simulink model "MPCsimulation_tuning_2016B"  (R2016b)
settings: Solver=VariableStepAuto  StartTime=0.0  StopTime=30.0  RelTol=1e-3
InitFcn:
  | dynrotpend
undefined symbols (not defined in the file or in its folder): matrcomp, par
libraries: dspinverses x2, mpclib x1, simulink x1
settings Model: Creator=janneke  LastModifiedBy=janneke
settings SFSimCC: SimUseLocalCustomCode=on
settings RTWCC: RTWUseLocalCustomCode=on

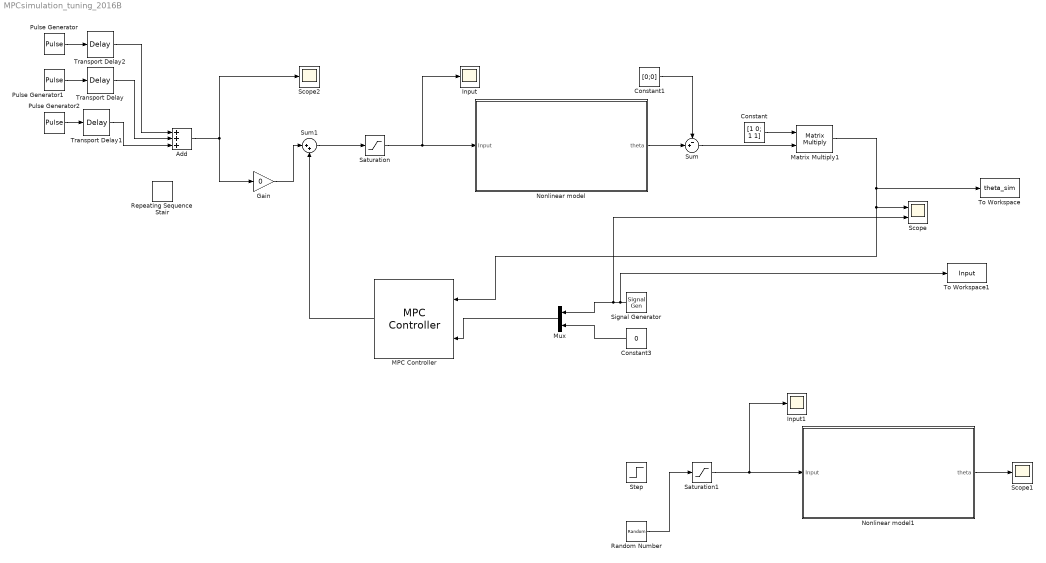
== system MPCsimulation_tuning_2016B ==
  Add : Sum  Inputs=+++
  Constant : Constant  Value=[1 0; 1 1]
  Constant1 : Constant  Value=[0;0]
  Constant3 : Constant  Value=0
  Gain : Gain  Gain=0
  Input : Scope
  Input1 : Scope
  MPC Controller : mpclib/MPC Controller  SCDEnableBlockLinearizationSpecification=on  mpcobj=MPCobj_tuning  is_multiple=0  enable_value=0  return_u0=off  updateMPCinCallerWorkspace=on  md_inport=off  mv_inport=off  cost_outport=off  return_sequence=off  return_qpstatus=off  return_xseq=off  return_state=off  return_ovseq=off  state_inport=off  umin_inport=off  umax_inport=off  ymin_inport=off  ymax_inport=off  cc_inport=off  ywt_inport=off  uwt_inport=off  duwt_inport=off  rhoeps_inport=off  uref_inport=off  n_ts=0.01  n_p=40  n_mv=1  n_md=0  n_ud=0  n_mo=2  n_uo=0  BlockDataType=double  SampleTimeInherited=off  switch_inport=off
  Matrix Multiply1 : Product  Multiplication=Matrix(*)
  Mux : Mux  Inputs=2
  Nonlinear model : Subsystem
  Nonlinear model1 : Subsystem
  Pulse Generator : DiscretePulseGenerator  PulseType=Time based  Amplitude=0.4  Period=10
  Pulse Generator1 : DiscretePulseGenerator  PulseType=Time based  Amplitude=0.2  Period=10
  Pulse Generator2 : DiscretePulseGenerator  PulseType=Time based  Amplitude=0.1  Period=10
  Random Number : RandomNumber  SampleTime=0.01
  Repeating Sequence Stair : simulink/Sources/Repeating Sequence Stair  OutValues=[0 0 0 0 0.4 zeros(1,15) 0.6 zeros(1,15) -0.8 zeros(1,11)].'  tsamp=0.1  OutMin=[]  OutMax=[]  OutDataTypeStr=double  OutputDataTypeScalingMode=double  OutDataType=fixdt(0,8)  ConRadixGroup=Best Precision: Vector-wise  OutScaling=2^-12
  Saturation : Saturate  UpperLimit=1  LowerLimit=-1
  Saturation1 : Saturate  UpperLimit=1  LowerLimit=-1
  Scope : Scope  NumInputPorts=2
  Scope1 : Scope
  Scope2 : Scope
  Signal Generator : SignalGenerator  Amplitude=0.4  Frequency=1/15
  Step : Step  Time=0  SampleTime=0
  Sum : Sum  Inputs=-+|
  Sum1 : Sum  Inputs=|++
  To Workspace : ToWorkspace  VariableName=theta_sim  SaveFormat=Timeseries  SampleTime=-1
  To Workspace1 : ToWorkspace  VariableName=Input  SaveFormat=Timeseries  SampleTime=-1
  Transport Delay : TransportDelay  DelayTime=15
  Transport Delay1 : TransportDelay  DelayTime=25
  Transport Delay2 : TransportDelay  DelayTime=5
  wires:
  Saturation/1 -> Input/1, Nonlinear model/1("Input ")
  MPC Controller/1 -> Sum1/2
  Constant/1 -> Matrix Multiply1/1
  Nonlinear model/1(theta) -> Sum/2
  Sum/1 -> Matrix Multiply1/2
  Constant1/1 -> Sum/1
  Mux/1 -> MPC Controller/2
  Constant3/1 -> Mux/2
  Signal Generator/1 -> To Workspace1/1, Scope/2, Mux/1
  Matrix Multiply1/1 -> To Workspace/1, MPC Controller/1, Scope/1
  Sum1/1 -> Saturation/1
  Nonlinear model1/1(theta) -> Scope1/1
  Saturation1/1 -> Input1/1, Nonlinear model1/1("Input ")
  Random Number/1 -> Saturation1/1
  Pulse Generator/1 -> Transport Delay2/1
  Pulse Generator1/1 -> Transport Delay/1
  Transport Delay/1 -> Add/2
  Add/1 -> Gain/1, Scope2/1
  Pulse Generator2/1 -> Transport Delay1/1
  Transport Delay1/1 -> Add/3
  Transport Delay2/1 -> Add/1
  Gain/1 -> Sum1/1

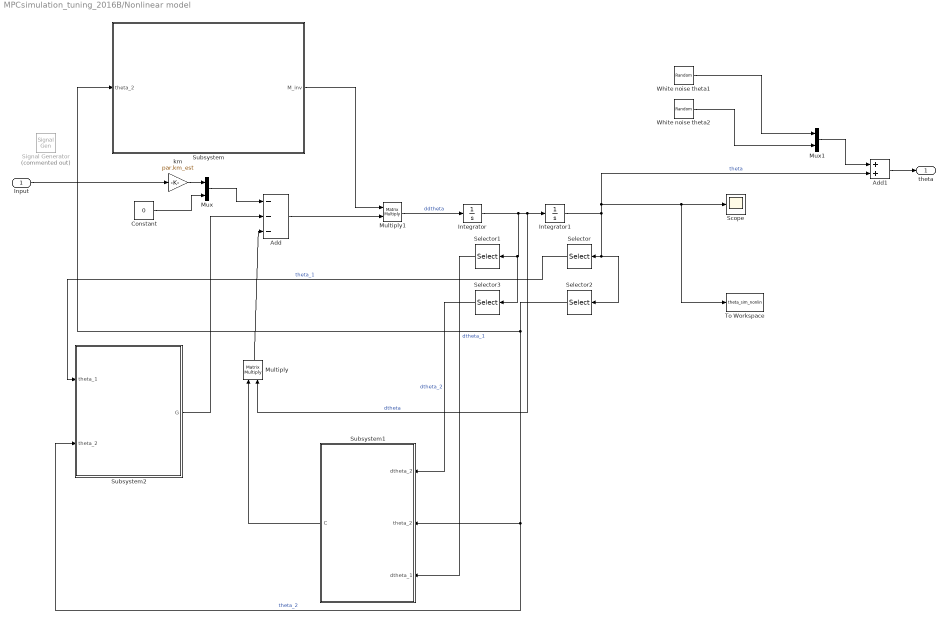
== system MPCsimulation_tuning_2016B/Nonlinear model ==
  "Input " : Inport
  Add : Sum  Inputs=---
  Add1 : Sum
  Constant : Constant  Value=0
  Integrator : Integrator  InitialCondition=[0;0]
  Integrator1 : Integrator  InitialCondition=[0;0]
  Multiply : Product  Multiplication=Matrix(*)
  Multiply1 : Product  Multiplication=Matrix(*)
  Mux : Mux  Inputs=2
  Mux1 : Mux  Inputs=2
  Scope : Scope
  Selector : Selector  InputPortWidth=2  IndexOptions=Index vector (dialog)  Indices=[1]  OutputSizes=1
  Selector1 : Selector  InputPortWidth=2  IndexOptions=Index vector (dialog)  Indices=[1]  OutputSizes=1
  Selector2 : Selector  InputPortWidth=2  IndexOptions=Index vector (dialog)  Indices=[2]  OutputSizes=1
  Selector3 : Selector  InputPortWidth=2  IndexOptions=Index vector (dialog)  Indices=[2]  OutputSizes=1
  Signal Generator : SignalGenerator  Commented=on  WaveForm=square  Amplitude=0.3
  Subsystem : Subsystem
  Subsystem1 : Subsystem
  Subsystem2 : Subsystem
  To Workspace : ToWorkspace  VariableName=theta_sim_nonlin  SaveFormat=Timeseries  SampleTime=-1
  "White noise theta1 " : RandomNumber  Variance=0.000001  SampleTime=0.1
  "White noise theta2 " : RandomNumber  Variance=0.00001  SampleTime=0.1
  km : Gain  Gain=par.km_est
  theta : Outport
  wires:
  "Input "/1 -> km/1
  Multiply/1 -> Add/3
  Subsystem2/1(G) -> Add/2
  Constant/1 -> Mux/2
  km/1 -> Mux/1
  Selector/1 -> Subsystem2/1(theta_1)  "theta_1"
  Subsystem/1(M_inv) -> Multiply1/1
  Subsystem1/1(C) -> Multiply/1
  Multiply1/1 -> Integrator/1  "ddtheta"
  Selector2/1 -> Subsystem2/2("theta_2 "), Subsystem1/2(theta_2), Subsystem/1("theta_2 ")  "theta_2"
  Add/1 -> Multiply1/2
  Mux/1 -> Add/1
  Selector1/1 -> Subsystem1/3(dtheta_1)  "dtheta_1"
  Integrator1/1 -> Add1/2, To Workspace/1, Scope/1, Selector2/1, Selector/1  "theta"
  Selector3/1 -> Subsystem1/1(dtheta_2)  "dtheta_2"
  Integrator/1 -> Multiply/2, Integrator1/1, Selector1/1, Selector3/1  "dtheta"
  "White noise theta1 "/1 -> Mux1/1
  "White noise theta2 "/1 -> Mux1/2
  Mux1/1 -> Add1/1
  Add1/1 -> theta/1

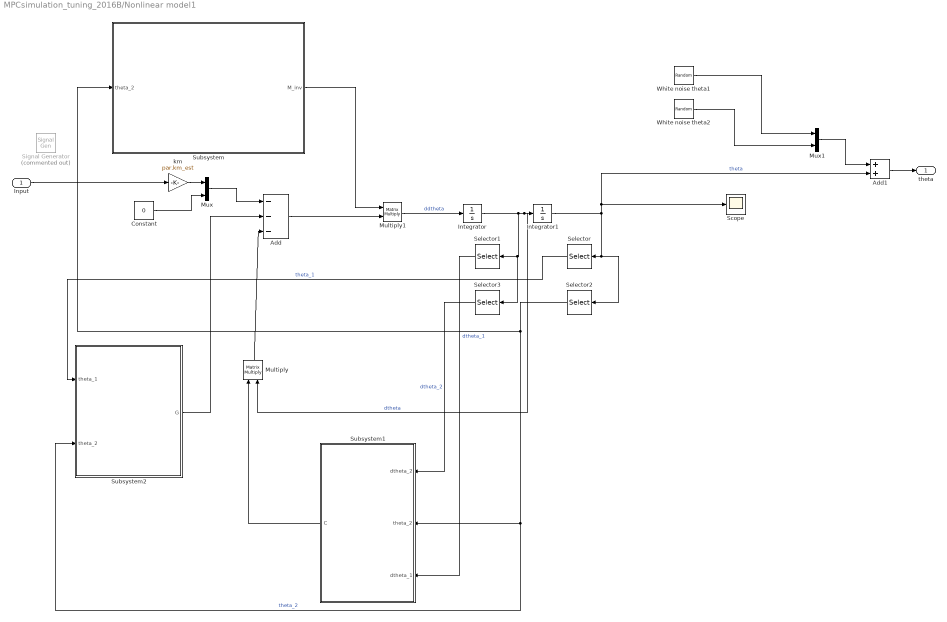
== system MPCsimulation_tuning_2016B/Nonlinear model1 ==
  "Input " : Inport
  Add : Sum  Inputs=---
  Add1 : Sum
  Constant : Constant  Value=0
  Integrator : Integrator  InitialCondition=[0;0]
  Integrator1 : Integrator  InitialCondition=[0;0]
  Multiply : Product  Multiplication=Matrix(*)
  Multiply1 : Product  Multiplication=Matrix(*)
  Mux : Mux  Inputs=2
  Mux1 : Mux  Inputs=2
  Scope : Scope
  Selector : Selector  InputPortWidth=2  IndexOptions=Index vector (dialog)  Indices=[1]  OutputSizes=1
  Selector1 : Selector  InputPortWidth=2  IndexOptions=Index vector (dialog)  Indices=[1]  OutputSizes=1
  Selector2 : Selector  InputPortWidth=2  IndexOptions=Index vector (dialog)  Indices=[2]  OutputSizes=1
  Selector3 : Selector  InputPortWidth=2  IndexOptions=Index vector (dialog)  Indices=[2]  OutputSizes=1
  Signal Generator : SignalGenerator  Commented=on  WaveForm=square  Amplitude=0.3
  Subsystem : Subsystem
  Subsystem1 : Subsystem
  Subsystem2 : Subsystem
  "White noise theta1 " : RandomNumber  Variance=6.7203e-06  SampleTime=0.1
  "White noise theta2 " : RandomNumber  Variance=1.3390e-5  SampleTime=0.1
  km : Gain  Gain=par.km_est
  theta : Outport
  wires:
  "Input "/1 -> km/1
  Multiply/1 -> Add/3
  Subsystem2/1(G) -> Add/2
  Constant/1 -> Mux/2
  km/1 -> Mux/1
  Selector/1 -> Subsystem2/1(theta_1)  "theta_1"
  Subsystem/1(M_inv) -> Multiply1/1
  Subsystem1/1(C) -> Multiply/1
  Multiply1/1 -> Integrator/1  "ddtheta"
  Selector2/1 -> Subsystem2/2("theta_2 "), Subsystem1/2(theta_2), Subsystem/1("theta_2 ")  "theta_2"
  Add/1 -> Multiply1/2
  Mux/1 -> Add/1
  Selector1/1 -> Subsystem1/3(dtheta_1)  "dtheta_1"
  Integrator1/1 -> Add1/2, Scope/1, Selector2/1, Selector/1  "theta"
  Selector3/1 -> Subsystem1/1(dtheta_2)  "dtheta_2"
  Integrator/1 -> Multiply/2, Integrator1/1, Selector1/1, Selector3/1  "dtheta"
  "White noise theta1 "/1 -> Mux1/1
  "White noise theta2 "/1 -> Mux1/2
  Mux1/1 -> Add1/1
  Add1/1 -> theta/1

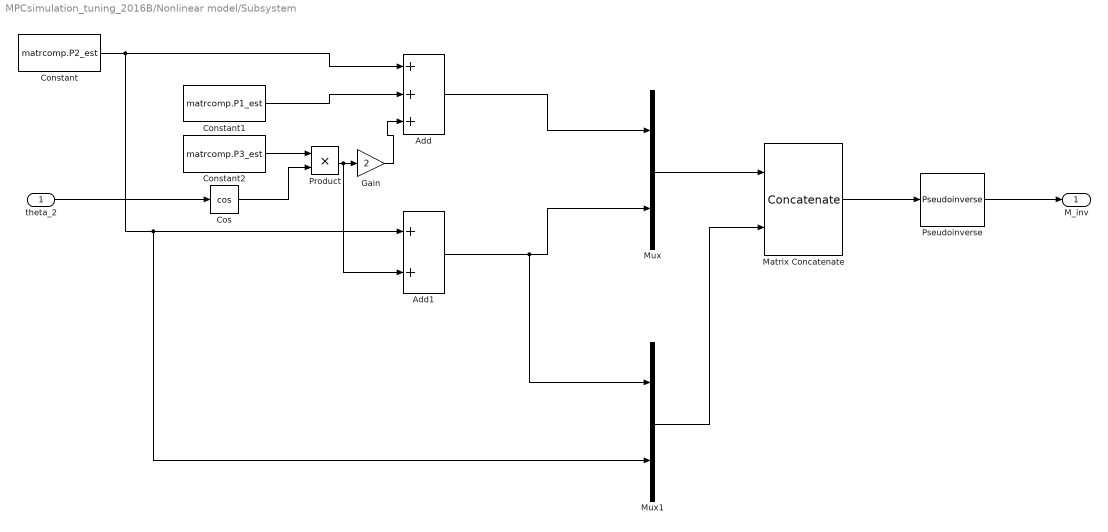
== system MPCsimulation_tuning_2016B/Nonlinear model/Subsystem ==
  "theta_2 " : Inport
  Add : Sum  Inputs=+++
  Add1 : Sum
  Constant : Constant  Value=matrcomp.P2_est
  Constant1 : Constant  Value=matrcomp.P1_est
  Constant2 : Constant  Value=matrcomp.P3_est
  Cos : Trigonometry  Operator=cos
  Gain : Gain  Gain=2
  Matrix Concatenate : Concatenate  Mode=Multidimensional array  ConcatenateDimension=2
  Mux : Mux  Inputs=2
  Mux1 : Mux  Inputs=2
  Product : Product
  Pseudoinverse : dspinverses/Pseudoinverse  wanterr=off  SimulateUsing=Interpreted execution
  M_inv : Outport
  wires:
  Product/1 -> Add1/2, Gain/1
  Mux/1 -> Matrix Concatenate/1
  Cos/1 -> Product/2
  "theta_2 "/1 -> Cos/1
  Gain/1 -> Add/3
  Constant1/1 -> Add/2
  Constant2/1 -> Product/1
  Mux1/1 -> Matrix Concatenate/2
  Matrix Concatenate/1 -> Pseudoinverse/1
  Pseudoinverse/1 -> M_inv/1
  Add/1 -> Mux/1
  Add1/1 -> Mux/2, Mux1/1
  Constant/1 -> Mux1/2, Add1/1, Add/1

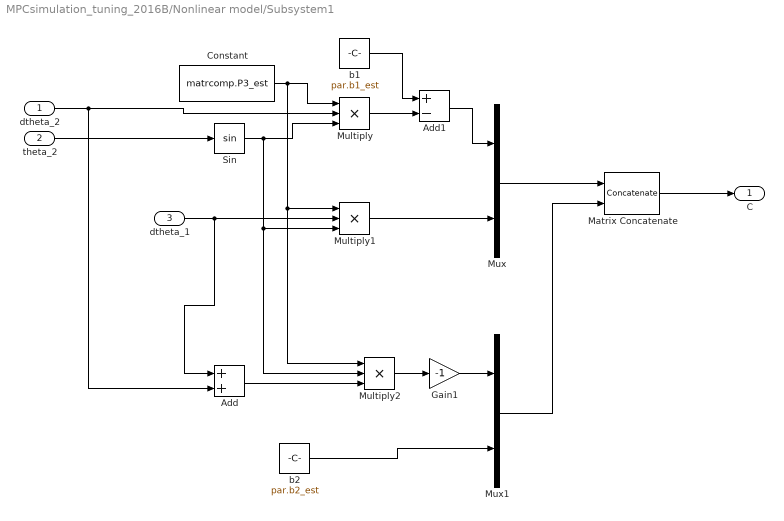
== system MPCsimulation_tuning_2016B/Nonlinear model/Subsystem1 ==
  dtheta_2 : Inport
  theta_2 : Inport  Port=2
  dtheta_1 : Inport  Port=3
  Add : Sum
  Add1 : Sum  Inputs=+-
  Constant : Constant  Value=matrcomp.P3_est
  Gain1 : Gain  Gain=-1
  Matrix Concatenate : Concatenate  Mode=Multidimensional array  ConcatenateDimension=2
  Multiply : Product  Inputs=3
  Multiply1 : Product  Inputs=3
  Multiply2 : Product  Inputs=3
  Mux : Mux  Inputs=2
  Mux1 : Mux  Inputs=2
  Sin : Trigonometry
  b1 : Constant  Value=par.b1_est
  b2 : Constant  Value=par.b2_est
  C : Outport
  wires:
  Gain1/1 -> Mux1/1
  Mux1/1 -> Matrix Concatenate/2
  Add/1 -> Multiply2/3
  Multiply2/1 -> Gain1/1
  dtheta_1/1 -> Add/1, Multiply1/2
  Multiply/1 -> Add1/2
  Matrix Concatenate/1 -> C/1
  Multiply1/1 -> Mux/2
  Constant/1 -> Multiply1/1, Multiply2/1, Multiply/1
  Mux/1 -> Matrix Concatenate/1
  b2/1 -> Mux1/2
  dtheta_2/1 -> Add/2, Multiply/2
  theta_2/1 -> Sin/1
  Sin/1 -> Multiply1/3, Multiply2/2, Multiply/3
  Add1/1 -> Mux/1
  b1/1 -> Add1/1

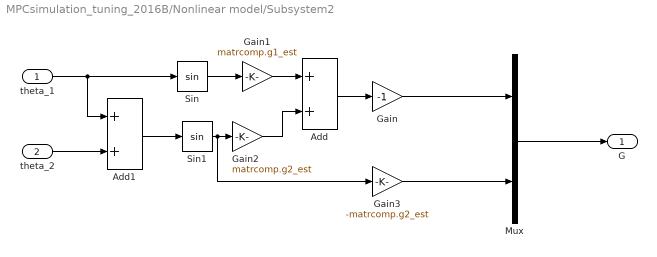
== system MPCsimulation_tuning_2016B/Nonlinear model/Subsystem2 ==
  theta_1 : Inport
  "theta_2 " : Inport  Port=2
  Add : Sum
  Add1 : Sum
  Gain : Gain  Gain=-1
  Gain1 : Gain  Gain=matrcomp.g1_est
  Gain2 : Gain  Gain=matrcomp.g2_est
  Gain3 : Gain  Gain=-matrcomp.g2_est
  Mux : Mux  Inputs=2
  Sin : Trigonometry
  Sin1 : Trigonometry
  G : Outport
  wires:
  Gain2/1 -> Add/2
  Mux/1 -> G/1
  Add1/1 -> Sin1/1
  Gain3/1 -> Mux/2
  Add/1 -> Gain/1
  Sin/1 -> Gain1/1
  Sin1/1 -> Gain3/1, Gain2/1
  Gain1/1 -> Add/1
  Gain/1 -> Mux/1
  "theta_2 "/1 -> Add1/2
  theta_1/1 -> Sin/1, Add1/1

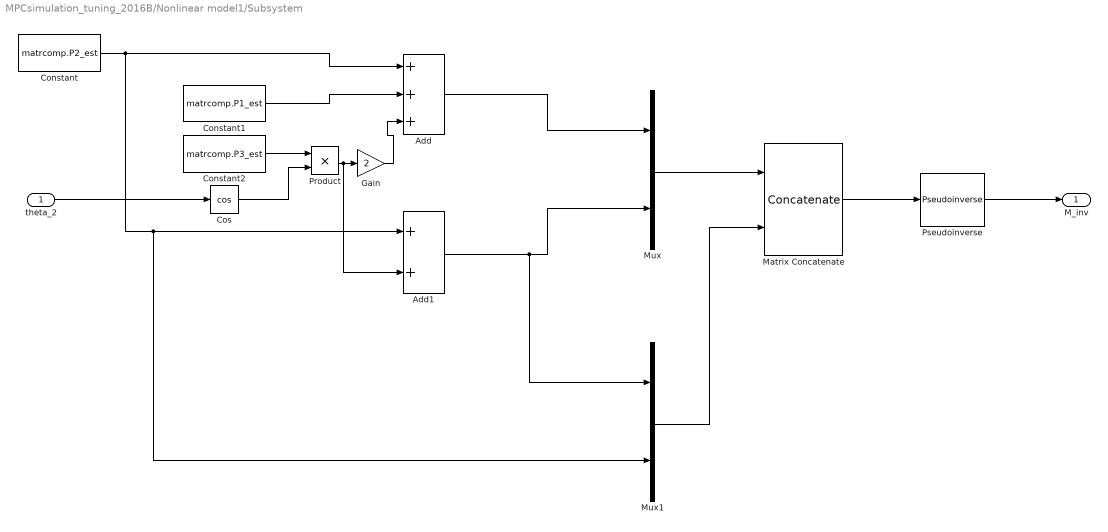
== system MPCsimulation_tuning_2016B/Nonlinear model1/Subsystem ==
  "theta_2 " : Inport
  Add : Sum  Inputs=+++
  Add1 : Sum
  Constant : Constant  Value=matrcomp.P2_est
  Constant1 : Constant  Value=matrcomp.P1_est
  Constant2 : Constant  Value=matrcomp.P3_est
  Cos : Trigonometry  Operator=cos
  Gain : Gain  Gain=2
  Matrix Concatenate : Concatenate  Mode=Multidimensional array  ConcatenateDimension=2
  Mux : Mux  Inputs=2
  Mux1 : Mux  Inputs=2
  Product : Product
  Pseudoinverse : dspinverses/Pseudoinverse  wanterr=off  SimulateUsing=Interpreted execution
  M_inv : Outport
  wires:
  Product/1 -> Add1/2, Gain/1
  Mux/1 -> Matrix Concatenate/1
  Cos/1 -> Product/2
  "theta_2 "/1 -> Cos/1
  Gain/1 -> Add/3
  Constant1/1 -> Add/2
  Constant2/1 -> Product/1
  Mux1/1 -> Matrix Concatenate/2
  Matrix Concatenate/1 -> Pseudoinverse/1
  Pseudoinverse/1 -> M_inv/1
  Add/1 -> Mux/1
  Add1/1 -> Mux/2, Mux1/1
  Constant/1 -> Mux1/2, Add1/1, Add/1

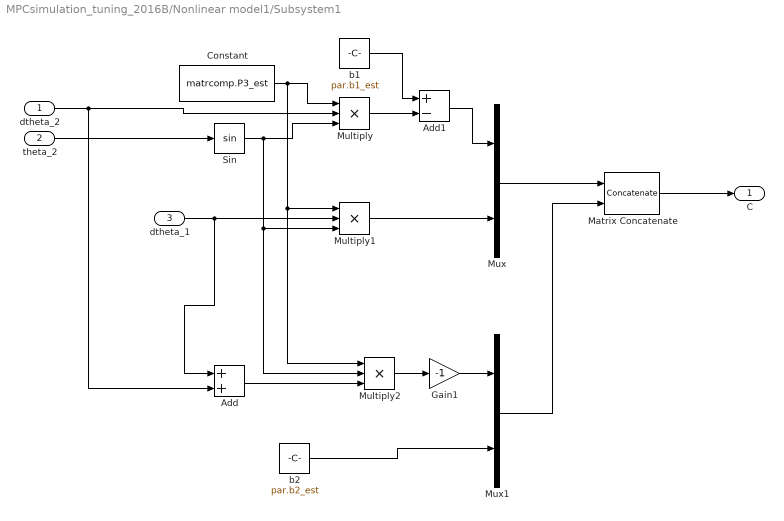
== system MPCsimulation_tuning_2016B/Nonlinear model1/Subsystem1 ==
  dtheta_2 : Inport
  theta_2 : Inport  Port=2
  dtheta_1 : Inport  Port=3
  Add : Sum
  Add1 : Sum  Inputs=+-
  Constant : Constant  Value=matrcomp.P3_est
  Gain1 : Gain  Gain=-1
  Matrix Concatenate : Concatenate  Mode=Multidimensional array  ConcatenateDimension=2
  Multiply : Product  Inputs=3
  Multiply1 : Product  Inputs=3
  Multiply2 : Product  Inputs=3
  Mux : Mux  Inputs=2
  Mux1 : Mux  Inputs=2
  Sin : Trigonometry
  b1 : Constant  Value=par.b1_est
  b2 : Constant  Value=par.b2_est
  C : Outport
  wires:
  Gain1/1 -> Mux1/1
  Mux1/1 -> Matrix Concatenate/2
  Add/1 -> Multiply2/3
  Multiply2/1 -> Gain1/1
  dtheta_1/1 -> Add/1, Multiply1/2
  Multiply/1 -> Add1/2
  Matrix Concatenate/1 -> C/1
  Multiply1/1 -> Mux/2
  Constant/1 -> Multiply1/1, Multiply2/1, Multiply/1
  Mux/1 -> Matrix Concatenate/1
  b2/1 -> Mux1/2
  dtheta_2/1 -> Add/2, Multiply/2
  theta_2/1 -> Sin/1
  Sin/1 -> Multiply1/3, Multiply2/2, Multiply/3
  Add1/1 -> Mux/1
  b1/1 -> Add1/1

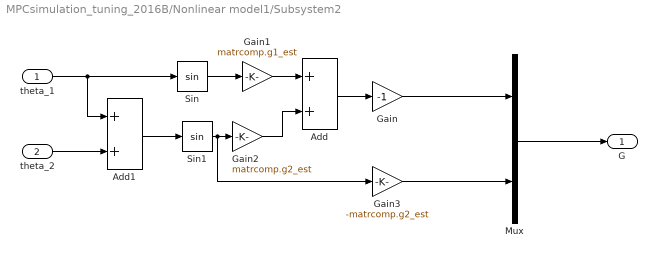
== system MPCsimulation_tuning_2016B/Nonlinear model1/Subsystem2 ==
  theta_1 : Inport
  "theta_2 " : Inport  Port=2
  Add : Sum
  Add1 : Sum
  Gain : Gain  Gain=-1
  Gain1 : Gain  Gain=matrcomp.g1_est
  Gain2 : Gain  Gain=matrcomp.g2_est
  Gain3 : Gain  Gain=-matrcomp.g2_est
  Mux : Mux  Inputs=2
  Sin : Trigonometry
  Sin1 : Trigonometry
  G : Outport
  wires:
  Gain2/1 -> Add/2
  Mux/1 -> G/1
  Add1/1 -> Sin1/1
  Gain3/1 -> Mux/2
  Add/1 -> Gain/1
  Sin/1 -> Gain1/1
  Sin1/1 -> Gain3/1, Gain2/1
  Gain1/1 -> Add/1
  Gain/1 -> Mux/1
  "theta_2 "/1 -> Add1/2
  theta_1/1 -> Sin/1, Add1/1
